simulink model "QuarterCar_Multibody"  (R2026a)
settings: Solver=ode15s  StopTime=20  MaxStep=1e-3  RelTol=1e-6
values from neighbouring files (symbols this model uses):
  m = P.mech    [build_quarter_car_multibody.m]    (also in build_quarter_car_simulink_v2.m; run_phase1.m = c10{i}.metrics; run_phase2.m = r.metrics; run_phase3.m = r.metrics)
  N = round(Pc.sim.T / Pc.sim.Ts)    [run_phase2.m]    (also in run_phase3.m = 40; run_quarter_car_replication.m = round(cfg.sim.duration_s / Ts))
  s = sprintf(fmt, v)    [run_phase1.m]    (also in run_phase2.m = ['MATLAB ', version])
libraries: nesl_utility x9, sm_lib x8
settings Model: Creator=Galaba Vamsi  LastModifiedBy=Galaba Vamsi

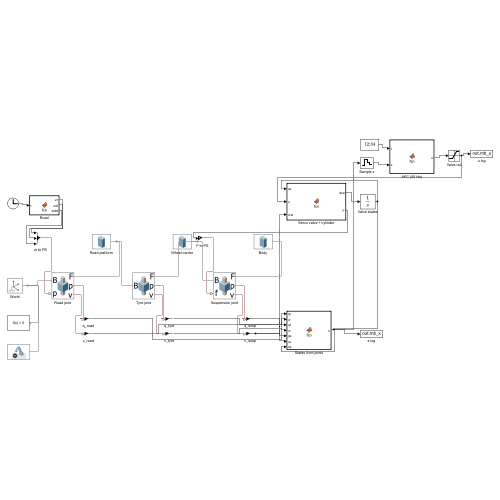
[thumbnail: Simulink's stored preview of the top-level diagram]
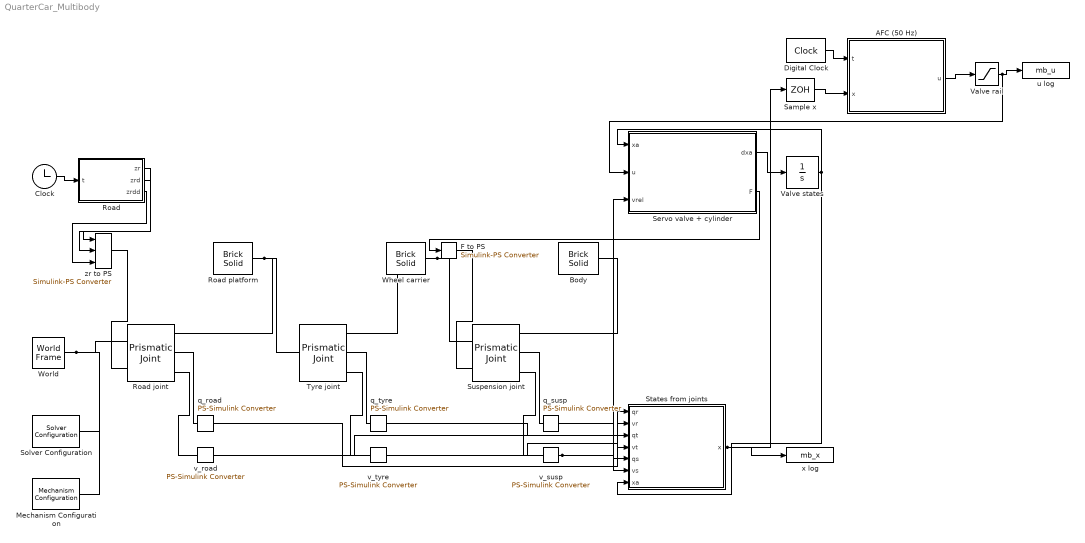
== system QuarterCar_Multibody ==
  AFC (50 Hz) : MATLAB Function  TreatAsAtomicUnit=on
  Body : sm_lib/Body Elements/Brick Solid  BrickDimensions=[0.86 0.42 0.13]  BrickDimensionsUnits=m  ExportEntireGeometry=off  InertiaType=CalculateFromGeometry  BasedOnType=Density  Density=6175.994548087571  DensityUnits=kg/m^3  Mass=1  MassUnits=kg  CenterOfMass=[0 0 0]  CenterOfMassUnits=m  MomentsOfInertia=[1 1 1]  MomentsOfInertiaUnits=kg*m^2  ProductsOfInertia=[0 0 0]  ProductsOfInertiaUnits=kg*m^2  GraphicType=FromGeometry  MarkerShape=Sphere  MarkerSize=10  GraphicVisPropType=SimpleVisualProperties  GraphicDiffuseColor=[0 0.4 0.5]  GraphicOpacity=1  GraphicSpecularColor=[0.5 0.5 0.5 1.0]  GraphicAmbientColor=[0.15 0.15 0.15 1.0]  GraphicEmissiveColor=[0.0 0.0 0.0 1.0]  GraphicShininess=75  DoExposeReferenceFrame=on  SerializedFrames=<Frames/>
  Clock : Clock
  Digital Clock : DigitalClock  SampleTime=0.02
  F to PS : nesl_utility/Simulink-PS Converter  PhysicalDomain=network_engine_domain  SubClassName=ps_input  LeftPortType=input  RightPortType=output  PseudoPeriodic=off  Frequencies=[]  NoiseDistribution=none  NoiseParameters=[]  Unit=N  AffineConversion=off  FilteringAndDerivatives=provide  SimscapeFilterOrder=1  InputFilterTimeConstant=0.001  UdotUserProvided=0
  Mechanism Configuration : sm_lib/Utilities/Mechanism Configuration  UniformGravity=None  GravityVector=[0 0 -9.80665]  GravityVectorUnits=m/s^2  LinearizationDelta=0.001  JointModeTransitionNonlinearIterations=2
  Road : MATLAB Function  TreatAsAtomicUnit=on
  Road joint : sm_lib/Joints/Prismatic Joint  JointMode=Normal  CompositeWrenchDir=FollowerOnBase  CompositeWrenchFrame=BaseFrame  SenseConstraintForce=off  SenseConstraintTorque=off  SenseTotalForce=off  SenseTotalTorque=off  PositionTargetSpecify=off  PositionTargetPriority=High  PositionTargetValue=0  PositionTargetValueUnits=m  VelocityTargetSpecify=off  VelocityTargetPriority=High  VelocityTargetValue=0  VelocityTargetValueUnits=m/s  EquilibriumPosition=0  EquilibriumPositionUnits=m  SpringStiffness=0  SpringStiffnessUnits=N/m  DampingCoefficient=0  DampingCoefficientUnits=N/(m/s)  LowerLimitSpecify=off  LowerLimitBound=-1  LowerLimitBoundUnits=m  LowerLimitStiffness=1e6  LowerLimitStiffnessUnits=N/m  LowerLimitDamping=1e3  LowerLimitDampingUnits=N/(m/s)  LowerLimitTransitionRegionWidth=1e-4  LowerLimitTransitionRegionWidthUnits=m  UpperLimitSpecify=off  UpperLimitBound=1  UpperLimitBoundUnits=m  UpperLimitStiffness=1e6  UpperLimitStiffnessUnits=N/m  UpperLimitDamping=1e3  UpperLimitDampingUnits=N/(m/s)  UpperLimitTransitionRegionWidth=1e-4  UpperLimitTransitionRegionWidthUnits=m  TorqueActuationMode=ComputedTorque  MotionActuationMode=InputMotion  SensePosition=on  SenseVelocity=on  SenseAcceleration=off  SenseTorqueForce=off  SenseLowerLimitTorqueForce=off  SenseUpperLimitTorqueForce=off
  Road platform : sm_lib/Body Elements/Brick Solid  BrickDimensions=[0.42 0.32 0.025]  BrickDimensionsUnits=m  ExportEntireGeometry=off  InertiaType=CalculateFromGeometry  BasedOnType=Density  Density=297.6190476190476  DensityUnits=kg/m^3  Mass=1  MassUnits=kg  CenterOfMass=[0 0 0]  CenterOfMassUnits=m  MomentsOfInertia=[1 1 1]  MomentsOfInertiaUnits=kg*m^2  ProductsOfInertia=[0 0 0]  ProductsOfInertiaUnits=kg*m^2  GraphicType=FromGeometry  MarkerShape=Sphere  MarkerSize=10  GraphicVisPropType=SimpleVisualProperties  GraphicDiffuseColor=[0.45 0.45 0.45]  GraphicOpacity=1  GraphicSpecularColor=[0.5 0.5 0.5 1.0]  GraphicAmbientColor=[0.15 0.15 0.15 1.0]  GraphicEmissiveColor=[0.0 0.0 0.0 1.0]  GraphicShininess=75  DoExposeReferenceFrame=on  SerializedFrames=<Frames/>
  Sample x : ZeroOrderHold  SampleTime=0.02
  Servo valve + cylinder : MATLAB Function  TreatAsAtomicUnit=on
  Solver Configuration : nesl_utility/Solver Configuration  PhysicalDomain=network_engine_domain  SubClassName=solver  LeftPortType=input  RightPortType=generic  Tones=[]  Harmonics=[]  SimulateNoise=off  Profile=off  UseLocalSampling=off  EnableSwitchedLinearOptims=on  FrequencyDomain=off  UseCCode=off  RelTol=0.001  AbsTol=0.001  MinStep=1e-09  ToWorkspace=off  RevertToSquareIcSolve=off  NumHomotopyIterations=100  PhasorMode=off  PhasorModeNumHarmonics=1  ConsistencySolver=NEWTON_XTOL_AFTER_FTOL  CanonicalOrdering=CANONICAL  OptimizeIntermediates=OPTIMIZED  IndexReductionMethod=DerivativeReplacement  DoDC=off  ResidualTolerance=1e-09  ConsistencyTolSource=GLOBAL  ConsistencyAbsTol=0.001  ConsistencyRelTol=0.001  ConsistencyTolFactor=0.001  UseLocalSolver=off  LocalSolverChoice=NE_BACKWARD_EULER_ADVANCER  ResolveIndetEquations=on  FunctionEvalNumThread=1  LocalSolverSampleTime=0.001  DoFixedCost=off  MaxNonlinIter=3  MaxModeIter=2  ComputeImpulses=off  ImpulseIterations=2  LinearAlgebra=auto  LinearAlgebraNumThread=0  EquationFormulation=NE_TIME_EF  DelaysMemoryBudget=1024  AutomaticFiltering=on  FilteringTimeConstant=0.001  PartitionStorageMethod=AS_NEEDED  PartitionMemoryBudget=1024  PartitionMethod=ROBUST  MultibodyUseLocalSolver=off  MultibodyLocalSolverChoice=ODE1  MultibodyLocalSolverSampleTime=0.001
  States from joints : MATLAB Function  TreatAsAtomicUnit=on
  Suspension joint : sm_lib/Joints/Prismatic Joint  JointMode=Normal  CompositeWrenchDir=FollowerOnBase  CompositeWrenchFrame=BaseFrame  SenseConstraintForce=off  SenseConstraintTorque=off  SenseTotalForce=off  SenseTotalTorque=off  PositionTargetSpecify=on  PositionTargetPriority=High  PositionTargetValue=0  PositionTargetValueUnits=m  VelocityTargetSpecify=on  VelocityTargetPriority=High  VelocityTargetValue=0  VelocityTargetValueUnits=m/s  EquilibriumPosition=0  EquilibriumPositionUnits=m  SpringStiffness=16812  SpringStiffnessUnits=N/m  DampingCoefficient=1000  DampingCoefficientUnits=N/(m/s)  LowerLimitSpecify=off  LowerLimitBound=-1  LowerLimitBoundUnits=m  LowerLimitStiffness=1e6  LowerLimitStiffnessUnits=N/m  LowerLimitDamping=1e3  LowerLimitDampingUnits=N/(m/s)  LowerLimitTransitionRegionWidth=1e-4  LowerLimitTransitionRegionWidthUnits=m  UpperLimitSpecify=off  UpperLimitBound=1  UpperLimitBoundUnits=m  UpperLimitStiffness=1e6  UpperLimitStiffnessUnits=N/m  UpperLimitDamping=1e3  UpperLimitDampingUnits=N/(m/s)  UpperLimitTransitionRegionWidth=1e-4  UpperLimitTransitionRegionWidthUnits=m  TorqueActuationMode=InputTorque  MotionActuationMode=ComputedMotion  SensePosition=on  SenseVelocity=on  SenseAcceleration=off  SenseTorqueForce=off  SenseLowerLimitTorqueForce=off  SenseUpperLimitTorqueForce=off
  Tyre joint : sm_lib/Joints/Prismatic Joint  JointMode=Normal  CompositeWrenchDir=FollowerOnBase  CompositeWrenchFrame=BaseFrame  SenseConstraintForce=off  SenseConstraintTorque=off  SenseTotalForce=off  SenseTotalTorque=off  PositionTargetSpecify=on  PositionTargetPriority=High  PositionTargetValue=0  PositionTargetValueUnits=m  VelocityTargetSpecify=on  VelocityTargetPriority=High  VelocityTargetValue=-0.1364393689454047  VelocityTargetValueUnits=m/s  EquilibriumPosition=0  EquilibriumPositionUnits=m  SpringStiffness=190000  SpringStiffnessUnits=N/m  DampingCoefficient=0  DampingCoefficientUnits=N/(m/s)  LowerLimitSpecify=off  LowerLimitBound=-1  LowerLimitBoundUnits=m  LowerLimitStiffness=1e6  LowerLimitStiffnessUnits=N/m  LowerLimitDamping=1e3  LowerLimitDampingUnits=N/(m/s)  LowerLimitTransitionRegionWidth=1e-4  LowerLimitTransitionRegionWidthUnits=m  UpperLimitSpecify=off  UpperLimitBound=1  UpperLimitBoundUnits=m  UpperLimitStiffness=1e6  UpperLimitStiffnessUnits=N/m  UpperLimitDamping=1e3  UpperLimitDampingUnits=N/(m/s)  UpperLimitTransitionRegionWidth=1e-4  UpperLimitTransitionRegionWidthUnits=m  TorqueActuationMode=NoTorque  MotionActuationMode=ComputedMotion  SensePosition=on  SenseVelocity=on  SenseAcceleration=off  SenseTorqueForce=off  SenseLowerLimitTorqueForce=off  SenseUpperLimitTorqueForce=off
  Valve rail : Saturate  UpperLimit=5  LowerLimit=-5
  Valve states : Integrator  InitialCondition=[0;0]
  Wheel carrier : sm_lib/Body Elements/Brick Solid  BrickDimensions=[0.82 0.11 0.06]  BrickDimensionsUnits=m  ExportEntireGeometry=off  InertiaType=CalculateFromGeometry  BasedOnType=Density  Density=10901.69992609017  DensityUnits=kg/m^3  Mass=1  MassUnits=kg  CenterOfMass=[0 0 0]  CenterOfMassUnits=m  MomentsOfInertia=[1 1 1]  MomentsOfInertiaUnits=kg*m^2  ProductsOfInertia=[0 0 0]  ProductsOfInertiaUnits=kg*m^2  GraphicType=FromGeometry  MarkerShape=Sphere  MarkerSize=10  GraphicVisPropType=SimpleVisualProperties  GraphicDiffuseColor=[0.3 0.45 0.6]  GraphicOpacity=1  GraphicSpecularColor=[0.5 0.5 0.5 1.0]  GraphicAmbientColor=[0.15 0.15 0.15 1.0]  GraphicEmissiveColor=[0.0 0.0 0.0 1.0]  GraphicShininess=75  DoExposeReferenceFrame=on  SerializedFrames=<Frames/>
  World : sm_lib/Frames and Transforms/World Frame
  q_road : nesl_utility/PS-Simulink Converter  PhysicalDomain=network_engine_domain  SubClassName=ps_output  LeftPortType=input  RightPortType=output  PseudoPeriodic=off  Frequencies=[]  VectorFormat=inherit  Unit=m  AffineConversion=off
  q_susp : nesl_utility/PS-Simulink Converter  PhysicalDomain=network_engine_domain  SubClassName=ps_output  LeftPortType=input  RightPortType=output  PseudoPeriodic=off  Frequencies=[]  VectorFormat=inherit  Unit=m  AffineConversion=off
  q_tyre : nesl_utility/PS-Simulink Converter  PhysicalDomain=network_engine_domain  SubClassName=ps_output  LeftPortType=input  RightPortType=output  PseudoPeriodic=off  Frequencies=[]  VectorFormat=inherit  Unit=m  AffineConversion=off
  u log : ToWorkspace  VariableName=mb_u  SaveFormat=Timeseries  SampleTime=-1
  v_road : nesl_utility/PS-Simulink Converter  PhysicalDomain=network_engine_domain  SubClassName=ps_output  LeftPortType=input  RightPortType=output  PseudoPeriodic=off  Frequencies=[]  VectorFormat=inherit  Unit=m/s  AffineConversion=off
  v_susp : nesl_utility/PS-Simulink Converter  PhysicalDomain=network_engine_domain  SubClassName=ps_output  LeftPortType=input  RightPortType=output  PseudoPeriodic=off  Frequencies=[]  VectorFormat=inherit  Unit=m/s  AffineConversion=off
  v_tyre : nesl_utility/PS-Simulink Converter  PhysicalDomain=network_engine_domain  SubClassName=ps_output  LeftPortType=input  RightPortType=output  PseudoPeriodic=off  Frequencies=[]  VectorFormat=inherit  Unit=m/s  AffineConversion=off
  x log : ToWorkspace  VariableName=mb_x  SaveFormat=Timeseries  SampleTime=-1
  zr to PS : nesl_utility/Simulink-PS Converter  PhysicalDomain=network_engine_domain  SubClassName=ps_input  LeftPortType=input  RightPortType=output  PseudoPeriodic=off  Frequencies=[]  NoiseDistribution=none  NoiseParameters=[]  Unit=m  AffineConversion=off  FilteringAndDerivatives=provide  SimscapeFilterOrder=1  InputFilterTimeConstant=0.001  UdotUserProvided=2
  wires:
  Clock/1 -> Road/1(t)
  Road/1(zr) -> zr to PS/1
  Road/2(zrd) -> zr to PS/2
  Road/3(zrdd) -> zr to PS/3
  q_road/1 -> States from joints/1(qr)
  v_road/1 -> States from joints/2(vr)
  q_tyre/1 -> States from joints/3(qt)
  v_tyre/1 -> States from joints/4(vt)
  q_susp/1 -> States from joints/5(qs)
  v_susp/1 -> States from joints/6(vs), Servo valve + cylinder/3(vrel)
  Valve states/1 -> States from joints/7(xa), Servo valve + cylinder/1(xa)
  Valve rail/1 -> Servo valve + cylinder/2(u), u log/1
  Servo valve + cylinder/1(dxa) -> Valve states/1
  Servo valve + cylinder/2(F) -> F to PS/1
  Digital Clock/1 -> AFC (50 Hz)/1(t)
  States from joints/1(x) -> Sample x/1, x log/1
  Sample x/1 -> AFC (50 Hz)/2(x)
  AFC (50 Hz)/1(u) -> Valve rail/1
  connections:
  Road joint/LConn1 -- World/RConn1 -- Solver Configuration/RConn1 -- Mechanism Configuration/RConn1
  Road platform/RConn1 -- Road joint/RConn1 -- Tyre joint/LConn1
  Wheel carrier/RConn1 -- Tyre joint/RConn1 -- Suspension joint/LConn1
  Suspension joint/RConn1 -- Body/RConn1
  zr to PS/RConn1 -- Road joint/LConn2
  F to PS/RConn1 -- Suspension joint/LConn2
  Road joint/RConn2 -- q_road/LConn1
  Road joint/RConn3 -- v_road/LConn1
  Tyre joint/RConn2 -- q_tyre/LConn1
  Tyre joint/RConn3 -- v_tyre/LConn1
  Suspension joint/RConn2 -- q_susp/LConn1
  Suspension joint/RConn3 -- v_susp/LConn1

== matlab function QuarterCar_Multibody/States from joints ==
  data: qr input; x output; vr input; qt input; vt input; qs input; vs input; xa input
function x = fcn(qr, vr, qt, vt, qs, vs, xa)
% series prismatic joints along Z: z_u = q_road + q_tyre, z_s = z_u + q_susp
x = zeros(6,1);
x(3) = qr + qt; x(4) = vr + vt;
x(1) = x(3) + qs; x(2) = x(4) + vs;
x(5) = xa(1); x(6) = xa(2);
end

== matlab function QuarterCar_Multibody/Road ==
  data: t input; zr output; zrd output; zrdd output
function [zr, zrd, zrdd] = fcn(t)
% paper road case 10: 0.043 m, 0.505 Hz
A = 0.043; w = 3.173008580125691;
zr = A*sin(w*t); zrd = A*w*cos(w*t); zrdd = -A*w^2*sin(w*t);
end

== matlab function QuarterCar_Multibody/Servo valve + cylinder ==
  data: xa input; u input; dxa output; vrel input; F output
function [dxa, F] = fcn(xa, u, vrel)
% Na et al. eqs. (2)-(6) with spool lag; xa = [x5; x_v], x5 = kappa*P_L
A=0.000335; alpha=45150000000000; beta=1; gamma=1545000000; Ps=10342500; kappa=1e-06; Kv=0.0005; tau=0.03333333333333333;
PL = xa(1)/kappa; xv = xa(2);
dPL = -beta*PL - alpha*A*vrel + gamma*xv*sqrt(max(Ps - sign(xv)*PL, 0));
dxa = [kappa*dPL; (Kv*u - xv)/tau];
F = A*PL;
end

== matlab function QuarterCar_Multibody/AFC (50 Hz) ==
  data: t input; u output; x input
function u = fcn(t, x)
mu0 = [0.2; 110; 100]; muinf = [0.018; 90; 80];
al = [3; 2; 2]; k = [25.5; 12; 216];
mu = (mu0 - muinf).*exp(-al*t) + muinf;
src = [x(1); x(2); x(5)]; prev = 0; v = 0;
for i = 1:3
  z = min(max((src(i) - prev)/mu(i), -1 + 1e-8), 1 - 1e-8);
  v = -k(i)*0.5*log((1 + z)/(1 - z)); prev = v;
end
u = v;
end
